simulink model "saturn_ib_stack_test"  (Simulink 6.2)
settings: Solver=ode4  SolverMode=SingleTasking  StartTime=-20.0  StopTime=620  FixedStep=0.005  RelTol=1e-3
values from neighbouring files (symbols this model uses):
  A_z_deg = 82.8200    (= 82.82)    [AS205_presettings.m]
  BN_1_sec = 14.4    [AS205_presettings.m]
  DeltaV_b_mps = 7.2381    [AS205_presettings.m]
  epsilon_2_sec = 15.0    (= 15)    [AS205_presettings.m]
  epsilon_prime_sec = 3.0    (= 3)    [AS205_presettings.m]
  i_deg = 28.89597    [AS205_presettings.m]
  lambda_0_deg = 102.32900    (= 102.329)    [AS205_presettings.m]
  lambda_L_deg = -80.561141    [AS205_presettings.m]
  pad_roll_L_deg = 100.0    (= 100)    [AS205_presettings.m]
  phi_L_deg = 28.521963    [AS205_presettings.m]
  phi_L_prime_deg = 28.360795    [AS205_presettings.m]
  R_L_m = 6373385.0    (= 6373385)    [AS205_presettings.m]
  R_T_m = 6570774.0    (= 6570774)    [AS205_presettings.m]
  T3_FM_sec = 6.08    [AS205_presettings.m]
  T_HSL_sec = 5.0    (= 5)    [AS205_presettings.m]
  Theta_T_deg = 0.000    (= 0)    [AS205_presettings.m]
  V_T_mps = 7780.976    [AS205_presettings.m]
  Xdotdot_VGT_mps2 = -9.251    [AS205_presettings.m]
undefined symbols (not defined in the file or in its folder): e0_0, e1_0, e2_0, e3_0, m, s
libraries: simulink x99, aerolibconvert x83, aerolibutil x63, aerolibtransform2 x34, aerolibasang x2, aerolibatmos2 x2, aerolib6dofsys x2
(part 3 of 7)

== system saturn_ib_stack_test/Saturn_IB_Stack/S-IB Stage/Retrorocket Motors ==
  note: This model does not account for possible
      | differences in individual rocket motor thrust.
  bRetroMotorStart : Inport  Port=1  LatchInput=off
  Angle Conversion : aerolibconvert/Angle Conversion  IU=deg  OU=rad
  Gain : Gain  Gain=-4.0
  Mux : Mux  Inputs=3
  Mux1 : Mux  Inputs=3
  Product : Product  RndMeth=Zero
  Retro Motor cant angle : Constant  Value=9.5
  S-IB Retrorocket Thrust : Lookup  InputValues=[0.0 0.02 0.1 0.7 1.0 1.1 1.2 1.4 1.46 1.6 1.8 2.70]  OutputValues="[0.0 170000 180000 172000 167000  160000 158000 157000 157000 75000 25000 0.0]"  LookUpMeth=Interpolation-Use End Values
  Switch : Switch  Criteria=u2 > Threshold  Threshold=0.0
  Time Since Engine Start : Subsystem
  Trigonometric Function : Trigonometry  Operator=cos
  zero : Constant  Value=0.0
  zero1 : Constant  Value=[ 0.0 0.0 0.0 ]
  Fb_N : Outport
  Mb_N : Outport  Port=2
  wires:
  Retro Motor cant angle/1 -> Angle Conversion/1
  Angle Conversion/1 -> Trigonometric Function/1
  Time Since Engine Start/1(T_elapsed_sec) -> S-IB Retrorocket Thrust/1
  bRetroMotorStart/1 -> Time Since Engine Start/1(bStart)
  S-IB Retrorocket Thrust/1 -> Gain/1, Switch/2
  zero/1 -> Mux/2, Mux/3, Mux1/1, Mux1/2, Mux1/3
  Gain/1 -> Product/1
  Trigonometric Function/1 -> Product/2
  Product/1 -> Mux/1
  Mux1/1 -> Mb_N/1
  Mux/1 -> Switch/1
  Switch/1 -> Fb_N/1
  zero1/1 -> Switch/3

== system saturn_ib_stack_test/Saturn_IB_Stack/S-IB Stage/Vehicle Mass Properties ==
  note: Vehicle C.G. relative to
      | STA. 100 (positive forward)
  note: These data taken from AS-205 Reference
      | Trajectory S-IB mass characteristics;
  note: Liftoff weight comes from AS-205 Revised
      | L/V Refernce Trajectory
  mdot_kg_per_sec : Inport  Port=1  LatchInput=off
  bStageSep : Inport  Port=2  DataType=boolean  LatchInput=off
  CG X : Lookup  InputValues=|  OutputValues=|
      InputValues=|
      | [179218
      | 179225
      | 180020
      | 182752
      | 185149
      | 196236
      | 210314
      | 224456
      | 238644
      | 252875
      | 267134
      | 281431
      | 295745
      | 310078
      | 324423
      | 338778
      | 353202
      | 367663
      | 382121
      | 396580
      | 411038
      | 425426
      | 439815
      | 454204
      | 468588
      | 482967
      | 497330
      | 511673
      | 525995
      | 540243
      | 554412
      | 568480
      | 582491]
      OutputValues=|
      | [25.1440
      | 25.1440
      | 25.0557
      | 24.7247
      | 24.4584
      | 23.3056
      | 22.0548
      | 20.9990
      | 20.0932
      | 19.3229
      | 18.6591
      | 18.0941
      | 17.6068
      | 17.1932
      | 16.8385
      | 16.5392
      | 16.2823
      | 16.0685
      | 15.8906
      | 15.7477
      | 15.6373
      | 15.5551
      | 15.4957
      | 15.4585
      | 15.4409
      | 15.4422
      | 15.4591
      | 15.4918
      | 15.5375
      | 15.5959
      | 15.6648
      | 15.7444
      | 15.8332]
  CG Y : Lookup  InputValues=|  OutputValues=|
      InputValues=|
      | [179218
      | 179225
      | 180020
      | 182752
      | 185149
      | 196236
      | 210314
      | 224456
      | 238644
      | 252875
      | 267134
      | 281431
      | 295745
      | 310078
      | 324423
      | 338778
      | 353202
      | 367663
      | 382121
      | 396580
      | 411038
      | 425426
      | 439815
      | 454204
      | 468588
      | 482967
      | 497330
      | 511673
      | 525995
      | 540243
      | 554412
      | 568480
      | 582491]
      OutputValues=|
      | [0.0021
      | 0.0021
      | 0.0206
      | 0.0203
      | 0.0201
      | 0.0191
      | 0.0178
      | 0.0165
      | 0.0155
      | 0.0147
      | 0.0140
      | 0.0132
      | 0.0124
      | 0.0121
      | 0.0114
      | 0.0109
      | 0.0104
      | 0.0100
      | 0.0097
      | 0.0094
      | 0.0091
      | 0.0086
      | 0.0084
      | 0.0081
      | 0.0079
      | 0.0076
      | 0.0074
      | 0.0072
      | 0.0071
      | 0.0069
      | 0.0066
      | 0.0065
      | 0.0064
      | ]
  CG Z : Lookup  InputValues=|  OutputValues=|
      InputValues=|
      | [179218
      | 179225
      | 180020
      | 182752
      | 185149
      | 196236
      | 210314
      | 224456
      | 238644
      | 252875
      | 267134
      | 281431
      | 295745
      | 310078
      | 324423
      | 338778
      | 353202
      | 367663
      | 382121
      | 396580
      | 411038
      | 425426
      | 439815
      | 454204
      | 468588
      | 482967
      | 497330
      | 511673
      | 525995
      | 540243
      | 554412
      | 568480
      | 582491]
      OutputValues=|
      | [-0.0079
      | -0.0079
      | -0.0079
      | -0.0076
      | -0.0076
      | -0.0070
      | -0.0066
      | -0.0062
      | -0.0058
      | -0.0055
      | -0.0051
      | -0.0050
      | -0.0046
      | -0.0044
      | -0.0043
      | -0.0041
      | -0.0038
      | -0.0037
      | -0.0036
      | -0.0034
      | -0.0033
      | -0.0032
      | -0.0030
      | -0.0028
      | -0.0028
      | -0.0028
      | -0.0028
      | -0.0025
      | -0.0025
      | -0.0025
      | -0.0025
      | -0.0023
      | -0.0023
      | ]
  Constant : Constant  Value=0.0
  Create 3x3 Matrix : aerolibutil/Create 3x3 Matrix
  Ixx : Lookup  InputValues=|  OutputValues=|
      InputValues=|
      | [179218
      | 179225
      | 180020
      | 182752
      | 185149
      | 196236
      | 210314
      | 224456
      | 238644
      | 252875
      | 267134
      | 281431
      | 295745
      | 310078
      | 324423
      | 338778
      | 353202
      | 367663
      | 382121
      | 396580
      | 411038
      | 425426
      | 439815
      | 454204
      | 468588
      | 482967
      | 497330
      | 511673
      | 525995
      | 540243
      | 554412
      | 568480
      | 582491]
      OutputValues=|
      | [42782
      | 42782
      | 43191
      | 44541
      | 45361
      | 50230
      | 50293
      | 62379
      | 68482
      | 74605
      | 80743
      | 86896
      | 93055
      | 99216
      | 105379
      | 111540
      | 117719
      | 123909
      | 130100
      | 136295
      | 142475
      | 148652
      | 154847
      | 161049
      | 167264
      | 173502
      | 179739
      | 185962
      | 192161
      | 198312
      | 204449
      | 210509
      | 216249
      | ]
  Iyy : Lookup  InputValues=|  OutputValues=|
      InputValues=|
      | [179218
      | 179225
      | 180020
      | 182752
      | 185149
      | 196236
      | 210314
      | 224456
      | 238644
      | 252875
      | 267134
      | 281431
      | 295745
      | 310078
      | 324423
      | 338778
      | 353202
      | 367663
      | 382121
      | 396580
      | 411038
      | 425426
      | 439815
      | 454204
      | 468588
      | 482967
      | 497330
      | 511673
      | 525995
      | 540243
      | 554412
      | 568480
      | 582491]
      OutputValues=|
      | [2817336
      | 2517336
      | 2854758
      | 2988393
      | 3097544
      | 3543473
      | 4013504
      | 4397718
      | 4716876
      | 4978079
      | 5193914
      | 5369698
      | 5513863
      | 5629776
      | 5723518
      | 5797431
      | 5856868
      | 5902608
      | 5938224
      | 5963453
      | 5985578
      | 5996581
      | 6005593
      | 6009655
      | 6014230
      | 6016490
      | 6020537
      | 6026361
      | 6032428
      | 6044729
      | 6055422
      | 6072821
      | 6094787
      | ]
  Izz : Lookup  InputValues=|  OutputValues=|
      InputValues=|
      | [179218
      | 179225
      | 180020
      | 182752
      | 185149
      | 196236
      | 210314
      | 224456
      | 238644
      | 252875
      | 267134
      | 281431
      | 295745
      | 310078
      | 324423
      | 338778
      | 353202
      | 367663
      | 382121
      | 396580
      | 411038
      | 425426
      | 439815
      | 454204
      | 468588
      | 482967
      | 497330
      | 511673
      | 525995
      | 540243
      | 554412
      | 568480
      | 582491]
      OutputValues=|
      | [2817336
      | 2517336
      | 2854758
      | 2988393
      | 3097544
      | 3543473
      | 4013504
      | 4397718
      | 4716876
      | 4978079
      | 5193914
      | 5369698
      | 5513863
      | 5629776
      | 5723518
      | 5797431
      | 5856868
      | 5902608
      | 5938224
      | 5963453
      | 5985578
      | 5996581
      | 6005593
      | 6009655
      | 6014230
      | 6016490
      | 6020537
      | 6026361
      | 6032428
      | 6044729
      | 6055422
      | 6072821
      | 6094787
      | ]
  Mux3 : Mux  Inputs=3
  Post-separation CG : Constant  Value=[279.488*0.0254 0.0 0.0]
  Post-separation Mass (approximate) : Constant  Value=42000.0
  Propellant Sensor Dry : simulink/Logic and Bit Operations/Compare To Constant  relop=<=  const=198488.9  LogicOutDataTypeMode=boolean  ZeroCross=off
  Switch : Switch  Criteria=u2 ~= 0
  Switch1 : Switch  Criteria=u2 ~= 0
  m_liftoff_kg : Constant  Value=586593.0
  vehicle mass (kg) : Integrator  InitialConditionSource=external
  m_kg : Outport
  Cg_m : Outport  Port=2
  I : Outport  Port=3
  bPropellant_Sensor_dry : Outport  Port=4
  wires:
  Ixx/1 -> Create 3x3 Matrix/1
  CG Y/1 -> Mux3/2
  CG X/1 -> Mux3/1
  CG Z/1 -> Mux3/3
  Create 3x3 Matrix/1 -> I/1  "I"
  Iyy/1 -> Create 3x3 Matrix/5
  Izz/1 -> Create 3x3 Matrix/9
  Constant/1 -> Create 3x3 Matrix/6, Create 3x3 Matrix/2, Create 3x3 Matrix/3, Create 3x3 Matrix/4, Create 3x3 Matrix/7, Create 3x3 Matrix/8
  vehicle mass (kg)/1 -> CG Z/1, CG Y/1, CG X/1, Izz/1, Ixx/1, Iyy/1, Propellant Sensor Dry/1, Switch1/3
  mdot_kg_per_sec/1 -> vehicle mass (kg)/1
  m_liftoff_kg/1 -> vehicle mass (kg)/2
  Propellant Sensor Dry/1 -> bPropellant_Sensor_dry/1
  Post-separation CG/1 -> Switch/1
  Switch/1 -> Cg_m/1
  Mux3/1 -> Switch/3  "Cg_m"
  bStageSep/1 -> Switch/2, Switch1/2
  Post-separation Mass (approximate)/1 -> Switch1/1
  Switch1/1 -> m_kg/1

== system saturn_ib_stack_test/Saturn_IB_Stack/S-IVB Stage/APS I Module ==
  note: Installation locations are approximate
  APS Relays : Inport  Port=1  LatchInput=off
  Cg_m : Inport  Port=2  LatchInput=off
  APS Thruster II : Subsystem  mask{r_m=[3.5 0.0 3.3], F_N=[0.0 670.0 0.0]}
      mask prompts: r_m "Installation Location (m)"; F_N "Thrust Vector (N)"
  APS Thruster IV : Subsystem  mask{r_m=[3.5 0.0 3.3], F_N=[0.0 -670.0 0.0]}
      mask prompts: r_m "Installation Location (m)"; F_N "Thrust Vector (N)"
  APS Thruster P : Subsystem  mask{r_m=[3.5 0.0 3.3], F_N=[0.0 0.0 -670.0]}
      mask prompts: r_m "Installation Location (m)"; F_N "Thrust Vector (N)"
  Demux : Demux  Outputs=3
  Sum : Sum  Inputs=+++
  Sum1 : Sum  Inputs=+++
  Fb_N : Outport
  Mb_Nm : Outport  Port=2
  wires:
  Sum1/1 -> Mb_Nm/1
  APS Thruster P/2(M_Nm) -> Sum1/2
  APS Thruster IV/2(M_Nm) -> Sum1/3
  APS Thruster II/1(F_N) -> Sum/1
  APS Thruster P/1(F_N) -> Sum/2
  Sum/1 -> Fb_N/1
  APS Thruster IV/1(F_N) -> Sum/3
  APS Thruster II/2(M_Nm) -> Sum1/1
  APS Relays/1 -> Demux/1
  Demux/3 -> APS Thruster IV/1(Fire)
  Cg_m/1 -> APS Thruster II/2(Cg_m), APS Thruster P/2(Cg_m), APS Thruster IV/2(Cg_m)
  Demux/2 -> APS Thruster II/1(Fire)
  Demux/1 -> APS Thruster P/1(Fire)

== system saturn_ib_stack_test/Saturn_IB_Stack/S-IVB Stage/APS III Module ==
  note: Installation locations are approximate
  APS Relays : Inport  Port=1  LatchInput=off
  Cg_m : Inport  Port=2  LatchInput=off
  APS Thruster II : Subsystem  mask{r_m=[3.5 0.0 -3.3], F_N=[0.0 670.0 0.0]}
      mask prompts: r_m "Installation Location (m)"; F_N "Thrust Vector (N)"
  APS Thruster IV : Subsystem  mask{r_m=[3.5 0.0 -3.3], F_N=[0.0 -670.0 0.0]}
      mask prompts: r_m "Installation Location (m)"; F_N "Thrust Vector (N)"
  APS Thruster P : Subsystem  mask{r_m=[3.5 0.0 -3.3], F_N=[0.0 0.0 670.0]}
      mask prompts: r_m "Installation Location (m)"; F_N "Thrust Vector (N)"
  Demux : Demux  Outputs=3
  Sum : Sum  Inputs=+++
  Sum1 : Sum  Inputs=+++
  Fb_N : Outport
  Mb_Nm : Outport  Port=2
  wires:
  Sum1/1 -> Mb_Nm/1
  APS Thruster P/2(M_Nm) -> Sum1/2
  APS Thruster IV/2(M_Nm) -> Sum1/3
  APS Thruster II/1(F_N) -> Sum/1
  APS Thruster P/1(F_N) -> Sum/2
  Sum/1 -> Fb_N/1
  APS Thruster IV/1(F_N) -> Sum/3
  APS Thruster II/2(M_Nm) -> Sum1/1
  APS Relays/1 -> Demux/1
  Demux/3 -> APS Thruster IV/1(Fire)
  Cg_m/1 -> APS Thruster P/2(Cg_m), APS Thruster IV/2(Cg_m), APS Thruster II/2(Cg_m)
  Demux/2 -> APS Thruster II/1(Fire)
  Demux/1 -> APS Thruster P/1(Fire)

== system saturn_ib_stack_test/Saturn_IB_Stack/S-IVB Stage/Aerodynamic Forces and Moments ==
  note: CP relative to Sta. 100 (positive forward)
  note: Aero forces at CP
  note: I am having a tough time finding NASA aero data for the
      | Saturn IB.  Use data from NASA-TM-X-53243 "Static Aerodynamic
      | Characteristics of the Aborted Saturn IB vehicle"
  note: C.G. relative to STA. 100
      | (positive forward)
  a_mps : Inport  Port=1  LatchInput=off
  rho : Inport  Port=2  LatchInput=off
  alpha_rad : Inport  Port=3  LatchInput=off
  beta_rad : Inport  Port=4  LatchInput=off
  V_mps : Inport  Port=5  LatchInput=off
  CG_m : Inport  Port=6  LatchInput=off
  3x3 Cross Product : aerolibutil/3x3 Cross Product
  Add : Sum  Inputs=+-|  OutScaling=2^-10
  Angle Conversion : aerolibconvert/Angle Conversion  IU=rad  OU=deg
  Angle Conversion1 : aerolibconvert/Angle Conversion  IU=rad  OU=deg
  CA_T : Lookup  InputValues=[0.0, 0.5, 0.75,1.0,1.25,1.5,6.0]  OutputValues=[1.2,0.84,0.74,0.96,1.02,0.95,0.48]
  CN(alpha) : Lookup2D  RowIndex=[0,0.2,0.4,1,2,3,4.8]  ColumnIndex=[0,2,4,6,8,10,12,14,15]  OutputValues=reshape([0.00,0.00,0.00,0.00,0,0,0,0.22,0.22,0.22,0.28,0.18,0.14,0.08,0.44,0.44,0.45,0.52,0.35,0.30,0.21,0.68,0.68,0.69,0.80,0.55,0.52,0.40,0.9,0.9,0.92,1.10,0.8,0.8,0.6,1.15,1.15,1.17,1.35,1.1,1.18,0.9,1.38,1.38,1.41,1.65,1.42,1.5,1.18,1.62,1.62,1.68,1.9,1.84,1.9,1.5,1.75,1.75,1.80,2.05,2.08,2.15,1.7],7,9)
  CN(beta) : Lookup2D  RowIndex=[0,0.2,0.4,1,2,3,4.8]  ColumnIndex=[0,2,4,6,8,10,12,14,15]  OutputValues=reshape([0.00,0.00,0.00,0.00,0,0,0,0.22,0.22,0.22,0.28,0.18,0.14,0.08,0.44,0.44,0.45,0.52,0.35,0.30,0.21,0.68,0.68,0.69,0.80,0.55,0.52,0.40,0.9,0.9,0.92,1.10,0.8,0.8,0.6,1.15,1.15,1.17,1.35,1.1,1.18,0.9,1.38,1.38,1.41,1.65,1.42,1.5,1.18,1.62,1.62,1.68,1.9,1.84,1.9,1.5,1.75,1.75,1.80,2.05,2.08,2.15,1.7],7,9)
  CP (m) : Lookup  InputValues=[0.0, 0.51, 1.2,1.54, 2.14, 6.28]  OutputValues=[17.95, 17.9109, 18.2259, 20.2936, 25.3718, 35.6068]
  Constant : Constant  Value=0.0
  Divide : Product  Inputs=*/  OutScaling=2^-10
  Dynamic Pressure : aerolibasang/Dynamic Pressure
  Mux : Mux  Inputs=3
  Mux1 : Mux  Inputs=3
  Product2 : Product  Inputs=3  RndMeth=Zero
  Referece Area (m^2) : Constant  Value=34.25
  Unary Minus : simulink/Math Operations/Unary Minus  DoSatur=off
  Unary Minus1 : simulink/Math Operations/Unary Minus  DoSatur=off
  Unary Minus2 : simulink/Math Operations/Unary Minus  DoSatur=off
  CP_m : Outport
  F_aero_N : Outport  Port=2
  M_aero_Nm : Outport  Port=3
  qbar : Outport  Port=4
  Mach : Outport  Port=5
  wires:
  V_mps/1 -> Divide/1, Dynamic Pressure/1
  Divide/1 -> CN(alpha)/1, CN(beta)/1, CA_T/1, Mach/1, CP (m)/1  "Mach Number"
  CN(alpha)/1 -> Unary Minus1/1
  CN(beta)/1 -> Unary Minus2/1
  CA_T/1 -> Unary Minus/1
  Mux/1 -> Product2/1
  Dynamic Pressure/1 -> Product2/2, qbar/1
  a_mps/1 -> Divide/2
  rho/1 -> Dynamic Pressure/2
  alpha_rad/1 -> Angle Conversion/1
  Product2/1 -> F_aero_N/1, 3x3 Cross Product/2
  beta_rad/1 -> Angle Conversion1/1
  Unary Minus/1 -> Mux/1
  CG_m/1 -> [CG_m]
  [CG_m] -> Add/2
  3x3 Cross Product/1 -> M_aero_Nm/1
  Add/1 -> 3x3 Cross Product/1
  CP (m)/1 -> Mux1/1
  Mux1/1 -> Add/1, CP_m/1
  Constant/1 -> Mux1/3, Mux1/2
  Referece Area (m^2)/1 -> Product2/3
  Unary Minus1/1 -> Mux/3
  Unary Minus2/1 -> Mux/2
  Angle Conversion/1 -> CN(alpha)/2
  Angle Conversion1/1 -> CN(beta)/2

== system saturn_ib_stack_test/Saturn_IB_Stack/S-IVB Stage/Custom Variable Mass 6DoF (Quaternion) ==
  Forces : Inport  Port=1  LatchInput=off
  Moments : Inport  Port=2  LatchInput=off
  m_dot : Inport  Port=3  LatchInput=off
  mass : Inport  Port=4  LatchInput=off
  I_dot : Inport  Port=5  LatchInput=off
  I : Inport  Port=6  LatchInput=off
  initial quaternion : Inport  Port=7  LatchInput=off
  Xe_initial_m : Inport  Port=8  PortDimensions=3  LatchInput=off
  Vb_0_mps : Inport  Port=9  LatchInput=off
  omega_0_rad_per_sec : Inport  Port=10  LatchInput=off
  Calculate DCM & Euler Angles : Subsystem  AncestorBlock=aerolib6dofsys/DCM & Euler Angles (Quaternion)
      mask Type: DCM & Euler Angles (Quaternion)
  Calculate omega_dot : Subsystem
  "Determine Force,  Mass & Inertia" : aerolib6dofsys/Mass & Inertia (custom)
  Out9 : Terminator
  Product : Product  Inputs=*/  SaturateOnIntegerOverflow=on
  Sum : Sum  Inputs=|++  SaturateOnIntegerOverflow=on
  Transpose : Math  Orientation=up  Operator=transpose  SaturateOnIntegerOverflow=on
  Vbxw : aerolibutil/3x3 Cross Product  Orientation=left
  Velocity Conversion : aerolibconvert/Velocity Conversion  IU=m/s  OU=m/s
  Velocity Conversion1 : aerolibconvert/Velocity Conversion  IU=m/s  OU=m/s
  "p,q,r " : Integrator  InitialConditionSource=external  InitialCondition=pm_0
  "transform to Inertial axes " : Subsystem
      mask Type: Vector Transformation
      mask Display: disp('L_EB')
  ub,vb,wb : Integrator  InitialConditionSource=external  InitialCondition=Vm_0
  xe,ye,ze : Integrator  InitialConditionSource=external  InitialCondition=xme_0
  Ve : Outport
  Xe : Outport  Port=2
  Euler : Outport  Port=3
  DCM : Outport  Port=4
  Vb : Outport  Port=5
  p,q,r : Outport  Port=6
  pdot,qdot,rdot : Outport  Port=7
  Ab : Outport  Port=8
  q : Outport  Port=9
  q0 : Outport  Port=10
  wires:
  Velocity Conversion1/1 -> Ve/1
  Velocity Conversion/1 -> Vb/1
  "Determine Force,  Mass & Inertia"/3 -> Calculate omega_dot/2("I, I_dot")
  Calculate DCM & Euler Angles/2(Euler) -> Euler/1
  Vbxw/1 -> Sum/2
  ub,vb,wb/1 -> Velocity Conversion/1, "transform to Inertial axes "/1(x y z), Vbxw/1, "Determine Force,  Mass & Inertia"/1
  Sum/1 -> ub,vb,wb/1
  xe,ye,ze/1 -> Xe/1
  "transform to Inertial axes "/1(Ve) -> Velocity Conversion1/1, xe,ye,ze/1
  "p,q,r "/1 -> p,q,r/1, Vbxw/2, Calculate omega_dot/1(p q r), Calculate DCM & Euler Angles/1(p q r)
  Moments/1 -> Calculate omega_dot/3(Moments)
  Forces/1 -> "Determine Force,  Mass & Inertia"/2
  Product/1 -> Sum/1, Ab/1
  Calculate DCM & Euler Angles/1(DCM) -> DCM/1, Transpose/1
  Transpose/1 -> "transform to Inertial axes "/2(transform coefficients)
  mass/1 -> "Determine Force,  Mass & Inertia"/3
  "Determine Force,  Mass & Inertia"/2 -> Product/2
  m_dot/1 -> "Determine Force,  Mass & Inertia"/4
  "Determine Force,  Mass & Inertia"/4 -> Out9/1
  Calculate omega_dot/1(pdot qdot rdot) -> pdot,qdot,rdot/1, "p,q,r "/1
  I/1 -> "Determine Force,  Mass & Inertia"/5
  I_dot/1 -> "Determine Force,  Mass & Inertia"/6
  "Determine Force,  Mass & Inertia"/1 -> Product/1
  Calculate DCM & Euler Angles/3(q) -> q/1
  initial quaternion/1 -> Calculate DCM & Euler Angles/2(Initial quaternion), q0/1
  Xe_initial_m/1 -> xe,ye,ze/2
  Vb_0_mps/1 -> ub,vb,wb/2
  omega_0_rad_per_sec/1 -> "p,q,r "/2

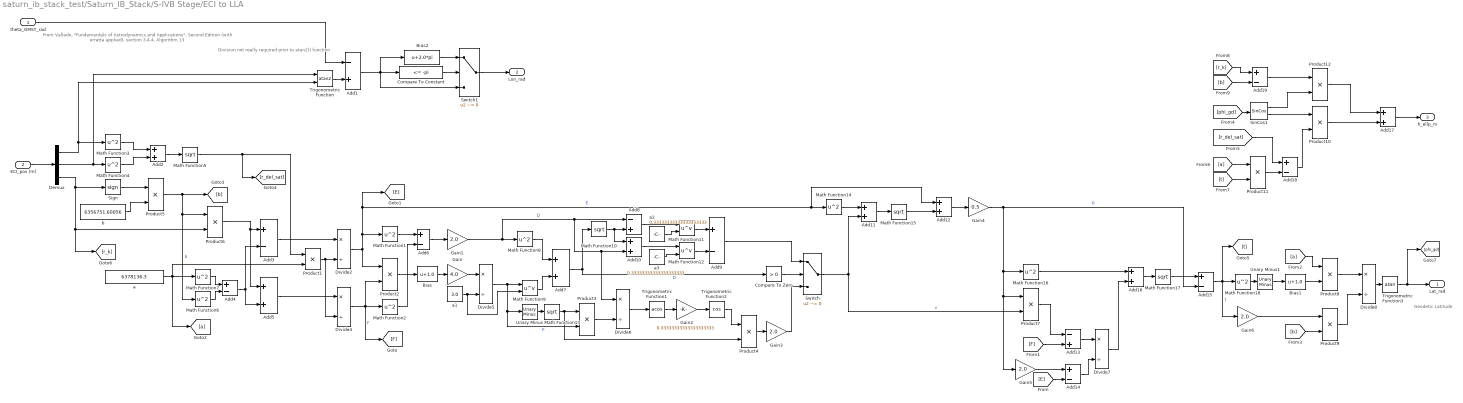
== system saturn_ib_stack_test/Saturn_IB_Stack/S-IVB Stage/ECI to LLA ==
  note: Division not really required
      | prior to atan2() function
  note: From Vallado, "Fundamentals of Astrodynamics and Applications",
      | Second Edition (with erratta applied), section 3.4.4, Algorithm 13
  note: Geodetic Latitude
  theta_GMST_rad : Inport  Port=1  LatchInput=off
  ECI_pos (m) : Inport  Port=2  LatchInput=off
  Add1 : Sum  Inputs=-+  OutScaling=2^-10
  Add{2,5,7,10..12,16..17} (8 alike) : Sum  OutScaling=2^-10
  Add13 : Sum  Inputs=-+  OutScaling=2^-10
  Add{3..4,6,9,14..15,18..19} (8 alike) : Sum  Inputs=+-  OutScaling=2^-10
  Add8 : Sum  Inputs=-+  OutScaling=2^-10
  Bias : Bias  Bias=1.0
  Bias1 : Bias  Bias=1.0
  Bias2 : Bias  Bias=2.0*pi
  Compare To Constant : simulink/Logic and Bit Operations/Compare To Constant  relop=<=  const=-pi  LogicOutDataTypeMode=boolean  ZeroCross=off
  Compare To Zero : simulink/Logic and Bit Operations/Compare To Zero  relop=>  LogicOutDataTypeMode=boolean  ZeroCross=off
  Demux : Demux  Outputs=3
  Divide{2,4..8} (6 alike) : Product  Inputs=*/  OutScaling=2^-10
  Gain : Gain  Gain=4.0
  Gain{1,3,5..6} (4 alike) : Gain  Gain=2.0
  Gain2 : Gain  Gain=0.33333333333333333333
  Gain4 : Gain  Gain=0.5
  Math Function{1..4,6..8,14,16,18} (10 alike) : Math  Operator=square  SaturateOnIntegerOverflow=on
  Math Function{5,10,13,15,17} (5 alike) : Math  Operator=sqrt  SaturateOnIntegerOverflow=on
  Math Function11 : Math  Operator=pow  SaturateOnIntegerOverflow=on
  Math Function12 : Math  Operator=pow  SaturateOnIntegerOverflow=on
  Math Function9 : Math  Operator=pow  SaturateOnIntegerOverflow=on
  Product{1..12} (12 alike) : Product  RndMeth=Zero
  Sign : Signum
  SinCos1 : aerolibutil/SinCos
  Switch : Switch  Criteria=u2 ~= 0
  Switch1 : Switch  Criteria=u2 ~= 0
  Trigonometric Function : Trigonometry  Operator=atan2
  Trigonometric Function1 : Trigonometry  Operator=acos
  Trigonometric Function2 : Trigonometry  Operator=cos
  Trigonometric Function3 : Trigonometry  Operator=atan
  Unary Minus : simulink/Math Operations/Unary Minus  DoSatur=off
  Unary Minus1 : simulink/Math Operations/Unary Minus  DoSatur=off
  a : Constant  Value=6378136.3  OutDataTypeMode=double
  a1 : Constant  Value=3.0  OutDataTypeMode=double
  a2 : Constant  Value=0.33333333333333333333  OutDataTypeMode=double
  a3 : Constant  Value=0.33333333333333333333  OutDataTypeMode=double
  b : Constant  Value=6356751.60056  OutDataTypeMode=double
  Lat_rad : Outport
  Lon_rad : Outport  Port=2
  h_ellp_m : Outport  Port=3
  wires:
  ECI_pos (m)/1 -> Demux/1
  Demux/1 -> Math Function3/1, Trigonometric Function/2
  Demux/2 -> Math Function4/1, Trigonometric Function/1
  Math Function3/1 -> Add2/1
  Math Function4/1 -> Add2/2
  Add2/1 -> Math Function5/1
  Demux/3 -> Sign/1, Product6/2, [r_k]
  Sign/1 -> Product5/1
  b/1 -> Product5/2
  Product5/1 -> Product6/1, Math Function6/1, [b]  "b"
  Product6/1 -> Add3/1, Add5/1
  Math Function6/1 -> Add4/2
  Math Function7/1 -> Add4/1
  a/1 -> Math Function7/1, Product1/2, [a]
  Add4/1 -> Add3/2, Add5/2
  Add3/1 -> Divide2/1
  Math Function5/1 -> Product1/1, [r_del_sat]
  Divide2/1 -> Product2/1, Math Function1/1, Math Function14/1, Add12/1, [E]  "E"
  Trigonometric Function/1 -> Add1/2
  theta_GMST_rad/1 -> Add1/1
  Product1/1 -> Divide2/2, Divide4/2
  Add5/1 -> Divide4/1
  Divide4/1 -> Product2/2, Math Function2/1, [F]  "F"
  Product2/1 -> Bias/1
  Bias/1 -> Gain/1
  Gain/1 -> Divide5/1
  a1/1 -> Divide5/2, Math Function9/2
  Divide5/1 -> Math Function9/1, Unary Minus/1, Product3/2  "P"
  Math Function1/1 -> Add6/1
  Math Function2/1 -> Add6/2
  Add6/1 -> Gain1/1
  Gain1/1 -> Math Function8/1, Add8/1, Add10/2, Divide6/1  "Q"
  Math Function8/1 -> Add7/1
  Math Function9/1 -> Add7/2
  Compare To Zero/1 -> Switch/2
  Add7/1 -> Compare To Zero/1, Math Function10/1  "D"
  Math Function10/1 -> Add8/2, Add10/1
  Add8/1 -> Math Function11/1
  a2/1 -> Math Function11/2
  Math Function11/1 -> Add9/1
  a3/1 -> Math Function12/2
  Math Function12/1 -> Add9/2
  Add10/1 -> Math Function12/1
  Add9/1 -> Switch/1
  Unary Minus/1 -> Math Function13/1
  Math Function13/1 -> Product3/1, Product4/2
  Product3/1 -> Divide6/2
  Divide6/1 -> Trigonometric Function1/1
  Trigonometric Function1/1 -> Gain2/1
  Gain2/1 -> Trigonometric Function2/1
  Trigonometric Function2/1 -> Product4/1
  Product4/1 -> Gain3/1
  Gain3/1 -> Switch/3
  Math Function14/1 -> Add11/1
  Switch/1 -> Add11/2, Product7/2  "v"
  Add11/1 -> Math Function15/1
  Math Function15/1 -> Add12/2
  Add12/1 -> Gain4/1
  Gain4/1 -> Math Function16/1, Product7/1, Gain5/1, Add15/2  "G"
  Product7/1 -> Add13/1
  [F] -> Add13/2
  Gain5/1 -> Add14/1
  [E] -> Add14/2
  Add13/1 -> Divide7/1
  Add14/1 -> Divide7/2
  Math Function16/1 -> Add16/1
  Divide7/1 -> Add16/2
  Add16/1 -> Math Function17/1
  Math Function17/1 -> Add15/1
  Add15/1 -> Math Function18/1, Gain6/1, [t]  "t"
  Math Function18/1 -> Unary Minus1/1
  Unary Minus1/1 -> Bias1/1
  Bias1/1 -> Product8/2
  [a] -> Product8/1
  Product8/1 -> Divide8/1
  Gain6/1 -> Product9/1
  Product9/1 -> Divide8/2
  [b] -> Product9/2
  Divide8/1 -> Trigonometric Function3/1
  Trigonometric Function3/1 -> Lat_rad/1, [phi_gd]
  [phi_gd] -> SinCos1/1
  Add17/1 -> h_ellp_m/1
  SinCos1/2 -> Product10/1
  [a] -> Product11/1
  [t] -> Product11/2
  Product11/1 -> Add18/2
  [r_del_sat] -> Add18/1
  Add18/1 -> Product10/2
  Product10/1 -> Add17/2
  [r_k] -> Add19/1
  [b] -> Add19/2
  Add19/1 -> Product12/1
  Product12/1 -> Add17/1
  SinCos1/1 -> Product12/2
  Add1/1 -> Compare To Constant/1, Bias2/1, Switch1/3
  Switch1/1 -> Lon_rad/1
  Compare To Constant/1 -> Switch1/2
  Bias2/1 -> Switch1/1

== system saturn_ib_stack_test/Saturn_IB_Stack/S-IVB Stage/Earth Gravity Model ==
  note: Gravity model accounts for Earth's oblateness.  From
      | Aircraft Control and Simulation, by Stevens and Lewis
      | who cite Brittling
  ECI_pos (m) : Inport  Port=1  PortDimensions=3  LatchInput=off
  theta_GMST_rad : Inport  Port=2  PortDimensions=1  LatchInput=off
  Add : Sum  Inputs=+++  OutScaling=2^-10
  Bias : Bias  Bias=3.0
  Bias1 : Bias  Bias=1.0
  Bias2 : Bias  Bias=1.0
  Demux : Demux  Outputs=3
  Divide : Product  Inputs=**/  OutScaling=2^-10
  Divide1 : Product  Inputs=*/  OutScaling=2^-10
  Divide2 : Product  Inputs=*/  OutScaling=2^-10
  GM : Constant  Value=3.986004418e14
  Gain : Gain  Gain=5.0
  Gain1 : Gain  Gain=1.5
  J1 : Constant  Value=3.0
  J2 : Constant  Value=0.00108263
  Math Function{,1..2,6} (4 alike) : Math  Operator=square  SaturateOnIntegerOverflow=on
  Math Function3 : Math  Operator=sqrt  SaturateOnIntegerOverflow=on
  Math Function5 : Math  Operator=pow  SaturateOnIntegerOverflow=on
  Mux : Mux  Inputs=3
  Product1 : Product  RndMeth=Zero
  Product3 : Product  Inputs=3  RndMeth=Zero
  Re : Constant  Value=6378137
  Terminator : Terminator
  Trigonometric Function : Trigonometry  Operator=asin
  Unary Minus : simulink/Math Operations/Unary Minus  DoSatur=off
  Unary Minus1 : simulink/Math Operations/Unary Minus  DoSatur=off
  g (m/s^2) : Outport  PortDimensions=3
  wires:
  ECI_pos (m)/1 -> Demux/1, Product1/2
  Demux/1 -> Math Function/1
  Demux/2 -> Math Function1/1
  Demux/3 -> Math Function2/1, Divide1/1
  Math Function/1 -> Add/1
  Math Function1/1 -> Add/2
  Math Function2/1 -> Add/3
  Add/1 -> Math Function3/1
  Divide1/1 -> Trigonometric Function/1
  Trigonometric Function/1 -> Gain/1
  Gain/1 -> Unary Minus1/1
  Unary Minus1/1 -> Bias1/1, Bias/1
  Re/1 -> Divide2/1
  Bias1/1 -> Mux/3, Mux/2
  Bias/1 -> Mux/1
  J2/1 -> Gain1/1
  Gain1/1 -> Product3/2
  Mux/1 -> Product3/3
  Divide2/1 -> Math Function6/1
  Math Function3/1 -> Divide2/2, Divide1/2, Math Function5/1
  GM/1 -> Divide/1
  Divide/1 -> Unary Minus/1
  Math Function5/1 -> Divide/3
  J1/1 -> Math Function5/2
  Unary Minus/1 -> g (m/s^2)/1
  Product3/1 -> Bias2/1
  Math Function6/1 -> Product3/1
  Bias2/1 -> Product1/1
  Product1/1 -> Divide/2
  theta_GMST_rad/1 -> Terminator/1

== system saturn_ib_stack_test/Saturn_IB_Stack/S-IVB Stage/J-2 Engine ==
  note: Individual engine performance estimates have been integrated
      | into this model.  See NASA-CR-95967 for the orignal values.
  CG_m : Inport  Port=1  LatchInput=off
  beta_P_deg : Inport  Port=2  LatchInput=off
  beta_Y_deg : Inport  Port=3  LatchInput=off
  bEngineCutoff : Inport  Port=4  PortDimensions=1  DataType=boolean  LatchInput=off
  bEngineStart : Inport  Port=5  PortDimensions=1  DataType=boolean  LatchInput=off
  Thrust Model : Subsystem
  Unary Minus : simulink/Math Operations/Unary Minus  DoSatur=off
  Fb_N : Outport
  Mb_Nm : Outport  Port=2
  mdot_kg_per_sec : Outport  Port=3
  wires:
  Thrust Model/3(mdot_kg_sec) -> Unary Minus/1
  beta_P_deg/1 -> Thrust Model/2(Pitch_actuator_cmd_deg)
  beta_Y_deg/1 -> Thrust Model/3(Yaw_actuator_cmd_deg)
  Thrust Model/1(F_N) -> Fb_N/1
  Thrust Model/2(M_Nm) -> Mb_Nm/1
  Unary Minus/1 -> mdot_kg_per_sec/1
  bEngineStart/1 -> Thrust Model/4(bEngineStart)
  bEngineCutoff/1 -> Thrust Model/5(bEngineCutoff)
  CG_m/1 -> Thrust Model/1(Cg_m)

== system saturn_ib_stack_test/Saturn_IB_Stack/S-IVB Stage/Relative Wind ==
  Xe_m : Inport  Port=1  LatchInput=off
  B_b : Inport  Port=2  LatchInput=off
  Vb_mps : Inport  Port=3  LatchInput=off
  3x3 Cross Product : aerolibutil/3x3 Cross Product
  "Incidence, Sideslip, & Airspeed" : Subsystem  AncestorBlock=aerolibasang/Incidence, Sideslip, & Airspeed
      mask Type: Incidence,Sideslip,&Airspeed
      mask Description: Calculate the angles between the body and the velocity vector (incidence and sideslip), and the velocity magnitude from the components in body axes (Vb).
      mask Help: web(asbhelp('incidence'));
      mask Display:
      | port_label('input',1,'V_b','texmode','on');
      | port_label('output',1,'\alpha','texmode','on');
      | port_label('output',2,'\beta','texmode','on');
      | port_label('output',3,'V','texmode','on');
  Product9 : Product  Multiplication=Matrix(*)  RndMeth=Zero
  Sum6 : Sum  Inputs=-+|
  omega_E_rad_per_sec : Constant  Value=[0.0 0.0 7.292115E-05]
  alpha_rad : Outport
  beta_rad : Outport  Port=2
  V_mps : Outport  Port=3
  wires:
  omega_E_rad_per_sec/1 -> 3x3 Cross Product/1
  3x3 Cross Product/1 -> Product9/2
  Sum6/1 -> "Incidence, Sideslip, & Airspeed"/1(Vb)
  Product9/1 -> Sum6/1
  B_b/1 -> Product9/1
  "Incidence, Sideslip, & Airspeed"/1(Alpha) -> alpha_rad/1
  "Incidence, Sideslip, & Airspeed"/2(Beta) -> beta_rad/1
  Vb_mps/1 -> Sum6/2
  "Incidence, Sideslip, & Airspeed"/3(V) -> V_mps/1
  Xe_m/1 -> 3x3 Cross Product/2

== system saturn_ib_stack_test/Saturn_IB_Stack/S-IVB Stage/Ullage Rocket Motors ==
  note: This model does not account for possible
      | differences in individual rocket motor thrust.
  bUllageMotorStart : Inport  Port=1  LatchInput=off
  Angle Conversion : aerolibconvert/Angle Conversion  IU=deg  OU=rad
  Gain : Gain  Gain=3.0
  Mux : Mux  Inputs=3
  Mux1 : Mux  Inputs=3
  Product : Product  RndMeth=Zero
  S-IVB Ullage Motor Thrust : Lookup  InputValues=[0.0 0.2 0.25 0.7 1.7 2.7 3.7 4.0 5.2 6.0 9.7]  OutputValues=[0.0 15500. 17000. 16500. 16300. 16200. 14500.0 9000.0 2500.0 1800. 0.0]  LookUpMeth=Interpolation-Use End Values
  Switch : Switch  Threshold=0.0
  Time Since Engine Start : Subsystem
  Trigonometric Function : Trigonometry  Operator=cos
  Ullage Motor cant angle : Constant  Value=35.0
  zero : Constant  Value=0.0
  Fb_N : Outport
  Mb_N : Outport  Port=2
  wires:
  Ullage Motor cant angle/1 -> Angle Conversion/1
  Angle Conversion/1 -> Trigonometric Function/1
  Time Since Engine Start/1(T_elapsed_sec) -> S-IVB Ullage Motor Thrust/1
  bUllageMotorStart/1 -> Time Since Engine Start/1(bStart)
  S-IVB Ullage Motor Thrust/1 -> Switch/2, Switch/1
  zero/1 -> Switch/3, Mux1/1, Mux/3, Mux/2, Mux1/3, Mux1/2
  Switch/1 -> Gain/1
  Gain/1 -> Product/1
  Trigonometric Function/1 -> Product/2
  Product/1 -> Mux/1
  Mux1/1 -> Mb_N/1
  Mux/1 -> Fb_N/1

== system saturn_ib_stack_test/Saturn_IB_Stack/S-IVB Stage/Vehicle Mass Properties ==
  note: Vehicle C.G. relative to
      | STA. 1086 (positive forward)
  note: These data taken from mass characteristics in [1]
  note: Separation weight comes from AS-205 Revised
      | L/V Reference Trajectory [1], Table 3A
  note: 30679 estimated cutoff mass
      | in simulated flight from [1]; 668.63 kg
      | of propellant remains at cutoff according
      | to [1], page 1.
  mdot_kg_per_sec : Inport  Port=1  LatchInput=off
  bUllageJettison : Inport  Port=2  LatchInput=off
  bLESJettison : Inport  Port=3  DataType=boolean  LatchInput=off
  CG X : Lookup  InputValues=|  OutputValues=|
      InputValues=|
      | [30679
      | 30680
      | 30768
      | 33383
      | 37429
      | 41455
      | 45517
      | 49647
      | 53949
      | 54630
      | 58719
      | 63592
      | 68474
      | 73349
      | 78223
      | 83102
      | 87977
      | 92857
      | 97731
      | 102607
      | 107484
      | 112361
      | 117240
      | 122120
      | 124558
      | 125318
      | 130828
      | 135700
      | 135898
      | 136955
      | 137000
      | 137659
      | 137853
      | 137883
      | ]
      OutputValues=|
      | [17.5931
      | 17.5926
      | 17.5479
      | 16.3594
      | 14.8766
      | 13.7122
      | 12.7645
      | 11.9749
      | 11.2929
      | 11.1950
      | 10.6636
      | 10.1311
      | 9.6860
      | 9.3113
      | 8.9933
      | 8.7211
      | 8.4874
      | 8.2865
      | 8.1142
      | 7.9640
      | 7.8369
      | 7.7273
      | 7.6347
      | 7.5571
      | 7.5236
      | 7.5140
      | 8.3239
      | 8.2453
      | 8.2425
      | 8.2453
      | 8.2170
      | 8.2160
      | 8.2160
      | 8.2160
      | ]
  CG Y : Lookup  InputValues=|  OutputValues=|
      InputValues=|
      | [30679
      | 30680
      | 30768
      | 33383
      | 37429
      | 41455
      | 45517
      | 49647
      | 53949
      | 54630
      | 58719
      | 63592
      | 68474
      | 73349
      | 78223
      | 83102
      | 87977
      | 92857
      | 97731
      | 102607
      | 107484
      | 112361
      | 117240
      | 122120
      | 124558
      | 125318
      | 130828
      | 135700
      | 135898
      | 136955
      | 137000
      | 137659
      | 137853
      | 137883
      | ]
      OutputValues=|
      | [-0.0968
      | -0.0968
      | -0.0966
      | -0.0891
      | -0.0796
      | -0.0719
      | -0.0657
      | -0.0605
      | -0.0557
      | -0.0551
      | -0.0513
      | -0.0474
      | -0.0441
      | -0.0414
      | -0.0389
      | -0.0366
      | -0.0347
      | -0.0331
      | -0.0314
      | -0.0300
      | -0.0286
      | -0.0276
      | -0.0266
      | -0.0256
      | -0.0250
      | -0.0249
      | -0.0238
      | -0.0229
      | -0.0229
      | -0.0228
      | -0.0226
      | -0.0226
      | -0.0226
      | -0.0226
      | ]
  CG Z : Lookup  InputValues=|  OutputValues=|
      InputValues=|
      | [30679
      | 30680
      | 30768
      | 33383
      | 37429
      | 41455
      | 45517
      | 49647
      | 53949
      | 54630
      | 58719
      | 63592
      | 68474
      | 73349
      | 78223
      | 83102
      | 87977
      | 92857
      | 97731
      | 102607
      | 107484
      | 112361
      | 117240
      | 122120
      | 124558
      | 125318
      | 130828
      | 135700
      | 135898
      | 136955
      | 137000
      | 137659
      | 137853
      | 137883
      | ]
      OutputValues=|
      | [-0.0328
      | -0.0328
      | -0.0327
      | -0.0301
      | -0.0269
      | -0.0242
      | -0.0219
      | -0.0201
      | -0.0184
      | -0.0183
      | -0.0169
      | -0.0156
      | -0.0144
      | -0.0134
      | -0.0126
      | -0.0118
      | -0.0112
      | -0.0106
      | -0.0101
      | -0.0096
      | -0.0090
      | -0.0086
      | -0.0083
      | -0.0079
      | -0.0078
      | -0.0076
      | -0.0078
      | -0.0074
      | -0.0074
      | -0.0074
      | -0.0074
      | -0.0074
      | -0.0074
      | -0.0074
      | ]
  Constant : Constant  Value=0.0
  Constant1 : Constant  Value=-8450.0  OutDataTypeMode=double
  Constant2 : Constant  Value=-220.0  OutDataTypeMode=double
  Create 3x3 Matrix : aerolibutil/Create 3x3 Matrix
  Ground : Ground
  Ixx : Lookup  InputValues=|  OutputValues=|
      InputValues=|
      | [30679
      | 30680
      | 30768
      | 33383
      | 37429
      | 41455
      | 45517
      | 49647
      | 53949
      | 54630
      | 58719
      | 63592
      | 68474
      | 73349
      | 78223
      | 83102
      | 87977
      | 92857
      | 97731
      | 102607
      | 107484
      | 112361
      | 117240
      | 122120
      | 124558
      | 125318
      | 130828
      | 135700
      | 135898
      | 136955
      | 137000
      | 137659
      | 137853
      | 137883
      | ]
      OutputValues=|
      | [13294
      | 13294
      | 13294
      | 13298
      | 13303
      | 13307
      | 13311
      | 13315
      | 13318
      | 13319
      | 13322
      | 13325
      | 13329
      | 13332
      | 13334
      | 13338
      | 13340
      | 13343
      | 13346
      | 13349
      | 13351
      | 13354
      | 13357
      | 13359
      | 13361
      | 13361
      | 13453
      | 13456
      | 13456
      | 13576
      | 13511
      | 13593
      | 13642
      | 13642
      | ]
  Iyy : Lookup  InputValues=|  OutputValues=|
      InputValues=|
      | [30679
      | 30680
      | 30768
      | 33383
      | 37429
      | 41455
      | 45517
      | 49647
      | 53949
      | 54630
      | 58719
      | 63592
      | 68474
      | 73349
      | 78223
      | 83102
      | 87977
      | 92857
      | 97731
      | 102607
      | 107484
      | 112361
      | 117240
      | 122120
      | 124558
      | 125318
      | 130828
      | 135700
      | 135898
      | 136955
      | 137000
      | 137659
      | 137853
      | 137883
      | ]
      OutputValues=|
      | [356888
      | 356912
      | 359090
      | 416336
      | 486596
      | 540625
      | 584100
      | 619892
      | 650469
      | 654832
      | 678390
      | 701074
      | 720881
      | 736855
      | 750242
      | 761591
      | 771303
      | 779584
      | 786634
      | 792844
      | 798039
      | 802626
      | 806568
      | 809927
      | 811425
      | 811860
      | 1119399
      | 1123582
      | 1123726
      | 1124798
      | 1125260
      | 1125364
      | 1125673
      | 1125673
      | ]
  Izz : Lookup  InputValues=|  OutputValues=|
      InputValues=|
      | [30679
      | 30680
      | 30768
      | 33383
      | 37429
      | 41455
      | 45517
      | 49647
      | 53949
      | 54630
      | 58719
      | 63592
      | 68474
      | 73349
      | 78223
      | 83102
      | 87977
      | 92857
      | 97731
      | 102607
      | 107484
      | 112361
      | 117240
      | 122120
      | 124558
      | 125318
      | 130828
      | 135700
      | 135898
      | 136955
      | 137000
      | 137659
      | 137853
      | 137883
      | ]
      OutputValues=|
      | [356888
      | 356912
      | 359090
      | 416336
      | 486596
      | 540625
      | 584100
      | 619892
      | 650469
      | 654832
      | 678390
      | 701674
      | 720881
      | 736855
      | 750242
      | 761591
      | 771303
      | 779584
      | 786634
      | 792844
      | 798039
      | 802626
      | 806568
      | 809927
      | 811425
      | 811860
      | 1119399
      | 1123582
      | 1123726
      | 1124798
      | 1125260
      | 1125364
      | 1125673
      | 1125673
      | ]
  Mass Conversion : aerolibconvert/Mass Conversion  IU=lbm  OU=kg
  Mass Conversion1 : aerolibconvert/Mass Conversion  IU=lbm  OU=kg
  Mux3 : Mux  Inputs=3
  Propellant Depleted : simulink/Logic and Bit Operations/Compare To Constant  relop=<  const=30074  LogicOutDataTypeMode=boolean  ZeroCross=off
  Subtract : Sum  Inputs=+++  OutScaling=2^-10
  Switch : Switch  Criteria=u2 ~= 0
  Switch1 : Switch  Criteria=u2 ~= 0
  m_separation_kg : Constant  Value=137883.0
  vehicle mass (kg) : Integrator  InitialConditionSource=external
  m_kg : Outport
  Cg_m : Outport  Port=2
  I : Outport  Port=3
  bPropellantDepleted : Outport  Port=4
  wires:
  Ixx/1 -> Create 3x3 Matrix/1
  CG X/1 -> Mux3/1
  Mux3/1 -> Cg_m/1  "Cg_m"
  Create 3x3 Matrix/1 -> I/1  "I"
  Iyy/1 -> Create 3x3 Matrix/5
  Izz/1 -> Create 3x3 Matrix/9
  Constant/1 -> Create 3x3 Matrix/6, Create 3x3 Matrix/2, Create 3x3 Matrix/3, Create 3x3 Matrix/4, Create 3x3 Matrix/7, Create 3x3 Matrix/8
  mdot_kg_per_sec/1 -> vehicle mass (kg)/1
  m_separation_kg/1 -> vehicle mass (kg)/2
  Propellant Depleted/1 -> bPropellantDepleted/1
  vehicle mass (kg)/1 -> Subtract/3
  Constant1/1 -> Mass Conversion/1
  bLESJettison/1 -> Switch/2
  Ground/1 -> Switch/3, Switch1/3
  Constant2/1 -> Mass Conversion1/1
  bUllageJettison/1 -> Switch1/2
  Switch/1 -> Subtract/2
  Switch1/1 -> Subtract/1
  Subtract/1 -> m_kg/1, Propellant Depleted/1, Iyy/1, Izz/1, Ixx/1, CG Z/1, CG Y/1, CG X/1
  CG Y/1 -> Mux3/2
  CG Z/1 -> Mux3/3
  Mass Conversion/1 -> Switch/1
  Mass Conversion1/1 -> Switch1/1

== system saturn_ib_stack_test/Saturn_IB_Stack/Saturn Instrument Unit (IU)/Accelerometers ==
  note: Sensor saturation
  A_b_mps2 : Inport  Port=1  LatchInput=off
  +/- 10 : Saturate  UpperLimit=10.0  LowerLimit=-10.0
  Constant : Constant  Value=0.0
  Demux2 : Demux  Outputs=2
  Mux1 : Mux  Inputs=3
  Selector : Selector  Elements=[3 2]  InputPortWidth=3
  Unary Minus : simulink/Math Operations/Unary Minus  DoSatur=off
  gamma_mps2 : Outport
  wires:
  Constant/1 -> Mux1/1
  Mux1/1 -> +/- 10/1
  +/- 10/1 -> gamma_mps2/1
  A_b_mps2/1 -> Selector/1
  Demux2/2 -> Unary Minus/1
  Selector/1 -> Demux2/1
  Demux2/1 -> Mux1/2
  Unary Minus/1 -> Mux1/3

== system saturn_ib_stack_test/Saturn_IB_Stack/Saturn Instrument Unit (IU)/Body Rate Gyros ==
  note: Gyro model from AS-203 document
  In1 : Inport  Port=1  LatchInput=off
  Angle Conversion : aerolibconvert/Angle Conversion  IU=rad  OU=deg
  Demux : Demux  Outputs=3
  Mux : Mux  Inputs=3
  Transfer Fcn : TransferFcn  Denominator=[6.333e-05 0.01114 1.0]
  Transfer Fcn1 : TransferFcn  Denominator=[6.333e-05 0.01114 1.0]
  Transfer Fcn2 : TransferFcn  Denominator=[6.333e-05 0.01114 1.0]
  sensor saturation : Saturate  UpperLimit=10.0  LowerLimit=-10.0
  phi_dot_deg_per_sec : Outport
  wires:
  In1/1 -> Angle Conversion/1
  sensor saturation/1 -> phi_dot_deg_per_sec/1
  Demux/2 -> Transfer Fcn1/1
  Demux/3 -> Transfer Fcn2/1
  Demux/1 -> Transfer Fcn/1
  Transfer Fcn/1 -> Mux/1
  Transfer Fcn1/1 -> Mux/2
  Transfer Fcn2/1 -> Mux/3
  Mux/1 -> sensor saturation/1
  Angle Conversion/1 -> Demux/1

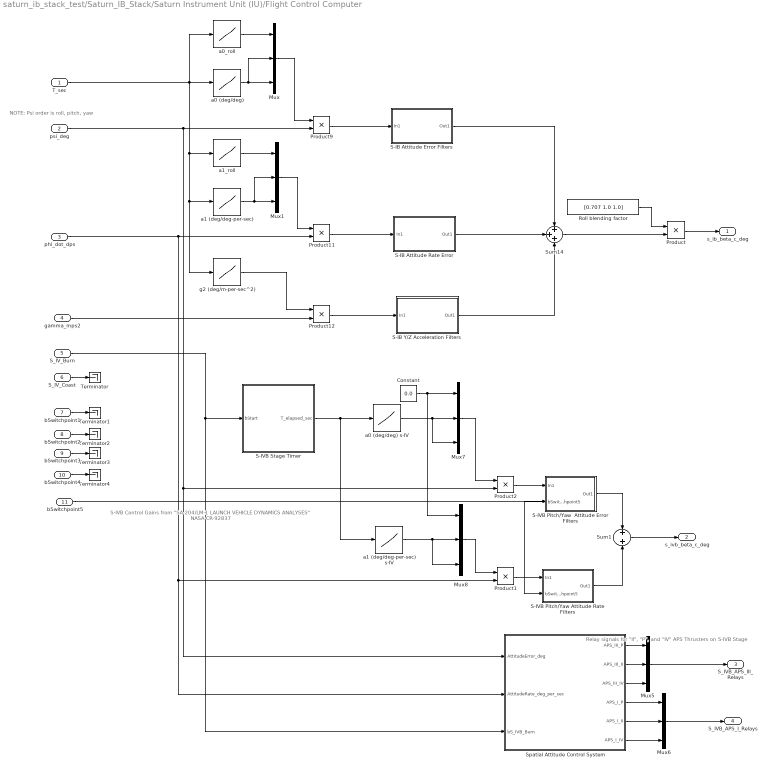
== system saturn_ib_stack_test/Saturn_IB_Stack/Saturn Instrument Unit (IU)/Flight Control Computer ==
  note: NOTE: Psi
      | order is roll, pitch, yaw
  note: Relay signals for "II", "P", and "IV"
      | APS Thrusters on S-IVB Stage
  note: S-IVB Control Gains from "SA-204/LM-1 LAUNCH
      | VEHICLE DYNAMICS ANALYSES"
      | NASA-CR-92837
  T_sec : Inport  Port=1  LatchInput=off
  psi_deg : Inport  Port=2  LatchInput=off
  phi_dot_dps : Inport  Port=3  LatchInput=off
  gamma_mps2 : Inport  Port=4  LatchInput=off
  S_IV_Burn : Inport  Port=5  LatchInput=off
  S_IV_Coast : Inport  Port=6  LatchInput=off
  bSwitchpoint1 : Inport  Port=7  LatchInput=off
  bSwitchpoint2 : Inport  Port=8  LatchInput=off
  bSwitchpoint3 : Inport  Port=9  LatchInput=off
  bSwitchpoint4 : Inport  Port=10  LatchInput=off
  bSwitchpoint5 : Inport  Port=11  LatchInput=off
  Constant : Constant  Value=0.0
  Mux{,1,5..8} (6 alike) : Mux  Inputs=3
  Product{,1..2,9,11..12} (6 alike) : Product  RndMeth=Zero
  Roll blending factor : Constant  Value=[0.707 1.0 1.0]
  S-IB Attitude Error Filters : Subsystem
  S-IB Attitude Rate Error : Subsystem
  S-IB Y/Z Acceleration Filters : Subsystem
  S-IVB Pitch/Yaw Attitude Rate Filters : Subsystem
  S-IVB Pitch/Yaw  Attitude Error Filters : Subsystem
  S-IVB Stage Timer : Subsystem
  Spatial Attitude Control System : Subsystem
  Sum1 : Sum  Inputs=+|+
  Sum14 : Sum  Inputs=+++
  Terminator{,1..4} (5 alike) : Terminator
  a0 (deg/deg) : Lookup  InputValues=[0.0 90.0 90.0 120.0 120.0 160.0]  OutputValues=[1.8 1.8 1.2 1.2 1.0 1.0]
  a0 (deg/deg) s-IV : Lookup  InputValues=[0.0 140.0 140.0 800.0]  OutputValues=[0.6 0.6 0.3 0.3]
  a0_roll : Lookup  InputValues=[0.0 40.0 40.0 100.0 100.0 160.0]  OutputValues=[0.30 0.30 0.23 0.23 0.15 0.15]
  a1 (deg/deg-per-sec) : Lookup  InputValues=[0.0 90.0 90.0 120.0 120.0 160.0]  OutputValues=[1.5 1.5 1.1 1.1 0.6 0.6]
  a1 (deg/deg-per-sec) s-IV : Lookup  InputValues=[0.0 140.0 140.0 800.0]  OutputValues=[0.4 0.4 0.2 0.2]
  a1_roll : Lookup  InputValues=[0.0 40.0 40.0 100.0 100.0 160.0 ]  OutputValues=[0.36 0.36 0.21 0.21 0.13 0.13]
  g2 (deg/m-per-sec^2) : Lookup  InputValues=[0.0 30.0 60.0 80.0 110.0 160.0]  OutputValues=[0.0 0.0 5.0 5.0 0.0 0.0]
  s_ib_beta_c_deg : Outport
  s_ivb_beta_c_deg : Outport  Port=2
  S_IVB_APS_III_Relays : Outport  Port=3  PortDimensions=3  DataType=boolean
  S_IVB_APS_I_Relays : Outport  Port=4  PortDimensions=3  DataType=boolean
  wires:
  g2 (deg/m-per-sec^2)/1 -> Product12/1
  T_sec/1 -> a0 (deg/deg)/1, a0_roll/1, g2 (deg/m-per-sec^2)/1, a1 (deg/deg-per-sec)/1, a1_roll/1
  psi_deg/1 -> Product9/2, Product2/2, Spatial Attitude Control System/1(AttitudeError_deg)
  phi_dot_dps/1 -> Product11/2, Product1/2, Spatial Attitude Control System/2(AttitudeRate_deg_per_sec)
  gamma_mps2/1 -> Product12/2
  a0_roll/1 -> Mux/1
  a0 (deg/deg)/1 -> Mux/2, Mux/3
  Mux/1 -> Product9/1
  a1 (deg/deg-per-sec)/1 -> Mux1/3, Mux1/2
  a1_roll/1 -> Mux1/1
  Mux1/1 -> Product11/1
  Roll blending factor/1 -> Product/1
  Sum14/1 -> Product/2
  Product/1 -> s_ib_beta_c_deg/1
  S-IB Attitude Error Filters/1(Out1) -> Sum14/1
  Product9/1 -> S-IB Attitude Error Filters/1(In1)
  Product12/1 -> S-IB Y/Z Acceleration Filters/1(In1)
  S-IB Y/Z Acceleration Filters/1(Out1) -> Sum14/3
  Spatial Attitude Control System/1(APS_III_P) -> Mux5/1
  Spatial Attitude Control System/2(APS_III_II) -> Mux5/2
  Spatial Attitude Control System/3(APS_III_IV) -> Mux5/3
  Spatial Attitude Control System/4(APS_I_P) -> Mux6/1
  Spatial Attitude Control System/5(APS_I_II) -> Mux6/2
  Spatial Attitude Control System/6(APS_I_IV) -> Mux6/3
  Mux5/1 -> S_IVB_APS_III_Relays/1
  Mux6/1 -> S_IVB_APS_I_Relays/1
  Mux8/1 -> Product1/1
  Mux7/1 -> Product2/1
  S_IV_Burn/1 -> S-IVB Stage Timer/1(bStart), Spatial Attitude Control System/3(bS_IVB_Burn)
  Product2/1 -> S-IVB Pitch/Yaw  Attitude Error Filters/1(In1)
  Sum1/1 -> s_ivb_beta_c_deg/1
  Constant/1 -> Mux7/1, Mux8/1
  S-IVB Pitch/Yaw  Attitude Error Filters/1(Out1) -> Sum1/1
  S_IV_Coast/1 -> Terminator/1
  bSwitchpoint1/1 -> Terminator1/1
  bSwitchpoint2/1 -> Terminator2/1
  bSwitchpoint3/1 -> Terminator3/1
  bSwitchpoint4/1 -> Terminator4/1
  bSwitchpoint5/1 -> S-IVB Pitch/Yaw  Attitude Error Filters/2(bSwitchpoint5), S-IVB Pitch/Yaw Attitude Rate Filters/2(bSwitchpoint5)
  S-IVB Pitch/Yaw Attitude Rate Filters/1(Out1) -> Sum1/2
  Product1/1 -> S-IVB Pitch/Yaw Attitude Rate Filters/1(In1)
  S-IVB Stage Timer/1(T_elapsed_sec) -> a0 (deg/deg) s-IV/1, a1 (deg/deg-per-sec) s-IV/1
  a0 (deg/deg) s-IV/1 -> Mux7/2, Mux7/3
  a1 (deg/deg-per-sec) s-IV/1 -> Mux8/2, Mux8/3
  Product11/1 -> S-IB Attitude Rate Error/1(In1)
  S-IB Attitude Rate Error/1(Out1) -> Sum14/2
